simulink model "bh_4bar_model_DYN"  (R2022b)
settings: Solver=ode45  StartTime=0.0  StopTime=10  FixedStep=0.001  MaxStep=0.1  RelTol=1e-9  AbsTol=1e-9  EnableMultiTasking=on
values from neighbouring files (symbols this model uses):
  L1 = 0.4    [bh_4bar_kin_z_analysis_CLS.m]
  L2 = 1.4    [bh_4bar_kin_z_analysis_CLS.m]
  L3 = 1.2    [bh_4bar_kin_z_analysis_CLS.m]
  L4 = 1    [bh_4bar_kin_z_analysis_CLS.m]
  N = length(THE_DEG_ANG_VEC)    [bh_4bar_kin_z_analysis_CLS.m]
  X = my_stuff_T.theta_deg_vec    [bh_4bar_kin_z_analysis_CLS.m]
undefined symbols (not defined in the file or in its folder): alpha_0_rad, alpha_dot_0_rad, alpha_rad, g, H, I_G1, I_G2, I_G3, m1, m2, m3, phi_0_rad, phi_dot_0_rad, phi_rad, theta_0_rad, theta_dot_0_rad, W, Y, Z
libraries: nesl_utility x20, sm_lib x15, simulink_extras x14, bh_4bar_SL_LIB x13
(part 3 of 3)

== matlab function bh_4bar_model_DYN/Hand_model_LAG_CONSTRAINTS_invA/THE_HAND_DYN_SYS1 ==
  data: I_1 input; theta_DD output; I_2 input; I_3 input; L_1 input; L_2 input; L_3 input; alpha input; alpha_dot input; g input; m_1 input; m_2 input; m_3 input; phi input; phi_dot input; tau_1 input; theta input; theta_dot input; alpha_DD output; phi_DD output; Lambda_1 output; Lambda_2 output
function [theta_DD,alpha_DD,phi_DD,Lambda_1,Lambda_2] = THE_HAND_DYN_SYS(I_1,I_2,I_3,L_1,L_2,L_3,alpha,alpha_dot,g,m_1,m_2,m_3,phi,phi_dot,tau_1,theta,theta_dot)
%#codegen

%    This function was generated by the Symbolic Math Toolbox version 8.4.
%    11-Nov-2019 10:59:12

theta_DD = (L_2.^2.*L_3.^2.*tau_1.*4.0-L_2.^2.*L_3.^2.*tau_1.*cos(alpha.*2.0-phi.*2.0).*4.0+I_3.*L_1.^2.*L_2.^2.*theta_dot.^2.*sin(alpha.*2.0-theta.*2.0).*4.0+I_2.*L_1.^2.*L_3.^2.*theta_dot.^2.*sin(phi.*2.0-theta.*2.0).*4.0+I_3.*L_1.*L_2.^3.*alpha_dot.^2.*sin(alpha-theta).*8.0-I_2.*L_1.*L_3.^3.*phi_dot.^2.*sin(phi-theta).*8.0+L_1.^2.*L_2.^2.*L_3.^2.*m_2.*theta_dot.^2.*sin(alpha.*2.0-theta.*2.0).*2.0+L_1.^2.*L_2.^2.*L_3.^2.*m_3.*theta_dot.^2.*sin(alpha.*2.0-theta.*2.0)-L_1.^2.*L_2.^2.*L_3.^2.*m_2.*theta_dot.^2.*sin(phi.*2.0-theta.*2.0)-I_2.*L_1.*L_2.*L_3.^2.*alpha_dot.^2.*sin(alpha-phi.*2.0+theta).*4.0+L_1.*L_2.^2.*L_3.^2.*g.*m_2.*cos(alpha.*2.0-theta)+L_1.*L_2.^2.*L_3.^2.*g.*m_3.*cos(alpha.*2.0-theta)+I_3.*L_1.*L_2.^2.*L_3.*phi_dot.^2.*sin(alpha.*-2.0+phi+theta).*4.0+L_1.*L_2.^3.*L_3.^2.*alpha_dot.^2.*m_2.*sin(alpha-theta).*3.0+L_1.*L_2.^3.*L_3.^2.*alpha_dot.^2.*m_3.*sin(alpha-theta).*2.0-L_1.*L_2.^2.*L_3.^2.*g.*m_2.*cos(phi.*2.0-theta)-L_1.*L_2.^2.*L_3.^2.*g.*m_3.*cos(phi.*2.0-theta)-L_1.*L_2.^2.*L_3.^3.*m_3.*phi_dot.^2.*sin(phi-theta)+L_1.*L_2.^2.*L_3.^2.*g.*m_1.*cos(alpha.*-2.0+phi.*2.0+theta)+L_1.*L_2.^2.*L_3.^2.*g.*m_1.*cos(alpha.*2.0-phi.*2.0+theta)+L_1.*L_2.^2.*L_3.^2.*g.*m_2.*cos(alpha.*-2.0+phi.*2.0+theta).*2.0+L_1.*L_2.^2.*L_3.^2.*g.*m_2.*cos(alpha.*2.0-phi.*2.0+theta)+L_1.*L_2.^2.*L_3.^2.*g.*m_3.*cos(alpha.*-2.0+phi.*2.0+theta)+L_1.*L_2.^3.*L_3.^2.*alpha_dot.^2.*m_2.*sin(alpha-phi.*2.0+theta)-L_1.*L_2.^2.*L_3.^2.*g.*m_1.*cos(theta).*2.0-L_1.*L_2.^2.*L_3.^2.*g.*m_2.*cos(theta).*3.0-L_1.*L_2.^2.*L_3.^2.*g.*m_3.*cos(theta)+I_2.*L_1.*L_2.*L_3.^2.*alpha_dot.^2.*sin(alpha-theta).*4.0+L_1.*L_2.^2.*L_3.^3.*m_2.*phi_dot.^2.*sin(alpha.*-2.0+phi+theta).*2.0+L_1.*L_2.^2.*L_3.^3.*m_3.*phi_dot.^2.*sin(alpha.*-2.0+phi+theta)-I_3.*L_1.*L_2.^2.*L_3.*phi_dot.^2.*sin(phi-theta).*4.0)./(I_1.*L_2.^2.*L_3.^2.*4.0+I_2.*L_1.^2.*L_3.^2.*4.0+I_3.*L_1.^2.*L_2.^2.*4.0-I_1.*L_2.^2.*L_3.^2.*cos(alpha.*2.0-phi.*2.0).*4.0-I_3.*L_1.^2.*L_2.^2.*cos(alpha.*2.0-theta.*2.0).*4.0-I_2.*L_1.^2.*L_3.^2.*cos(phi.*2.0-theta.*2.0).*4.0+L_1.^2.*L_2.^2.*L_3.^2.*m_1+L_1.^2.*L_2.^2.*L_3.^2.*m_2.*3.0+L_1.^2.*L_2.^2.*L_3.^2.*m_3-L_1.^2.*L_2.^2.*L_3.^2.*m_1.*cos(alpha.*2.0-phi.*2.0)-L_1.^2.*L_2.^2.*L_3.^2.*m_2.*cos(alpha.*2.0-phi.*2.0).*2.0-L_1.^2.*L_2.^2.*L_3.^2.*m_2.*cos(alpha.*2.0-theta.*2.0).*2.0-L_1.^2.*L_2.^2.*L_3.^2.*m_3.*cos(alpha.*2.0-theta.*2.0)+L_1.^2.*L_2.^2.*L_3.^2.*m_2.*cos(phi.*2.0-theta.*2.0));
if nargout > 1
    alpha_DD = -(L_1.*L_2.*L_3.^2.*tau_1.*cos(alpha-theta).*4.0+I_1.*L_2.^2.*L_3.^2.*alpha_dot.^2.*sin(alpha.*2.0-phi.*2.0).*4.0+I_3.*L_1.^2.*L_2.^2.*alpha_dot.^2.*sin(alpha.*2.0-theta.*2.0).*4.0-I_1.*L_2.*L_3.^3.*phi_dot.^2.*sin(alpha-phi).*8.0+I_3.*L_1.^3.*L_2.*theta_dot.^2.*sin(alpha-theta).*8.0-L_1.*L_2.*L_3.^2.*tau_1.*cos(alpha-phi.*2.0+theta).*4.0-I_3.*L_1.^2.*L_2.*L_3.*phi_dot.^2.*sin(alpha+phi-theta.*2.0).*4.0+I_1.*L_1.*L_2.*L_3.^2.*theta_dot.^2.*sin(alpha-phi.*2.0+theta).*4.0-L_1.^2.*L_2.*L_3.^3.*m_1.*phi_dot.^2.*sin(alpha-phi).*2.0-L_1.^2.*L_2.*L_3.^3.*m_2.*phi_dot.^2.*sin(alpha-phi).*6.0-L_1.^2.*L_2.*L_3.^3.*m_3.*phi_dot.^2.*sin(alpha-phi)+L_1.^3.*L_2.*L_3.^2.*m_1.*theta_dot.^2.*sin(alpha-theta)+L_1.^3.*L_2.*L_3.^2.*m_2.*theta_dot.^2.*sin(alpha-theta).*6.0+L_1.^3.*L_2.*L_3.^2.*m_3.*theta_dot.^2.*sin(alpha-theta).*2.0-L_1.^2.*L_2.*L_3.^2.*g.*m_1.*cos(alpha)+L_1.^2.*L_2.*L_3.^2.*g.*m_3.*cos(alpha)+L_1.^2.*L_2.*L_3.^2.*g.*m_1.*cos(alpha-phi.*2.0+theta.*2.0)+L_1.^2.*L_2.*L_3.^2.*g.*m_2.*cos(alpha-phi.*2.0+theta.*2.0)-L_1.^2.*L_2.*L_3.^2.*g.*m_2.*cos(alpha+phi.*2.0-theta.*2.0)-L_1.^2.*L_2.*L_3.^2.*g.*m_3.*cos(alpha+phi.*2.0-theta.*2.0)-L_1.^2.*L_2.*L_3.^3.*m_2.*phi_dot.^2.*sin(alpha+phi-theta.*2.0).*2.0-L_1.^2.*L_2.*L_3.^3.*m_3.*phi_dot.^2.*sin(alpha+phi-theta.*2.0)+L_1.^3.*L_2.*L_3.^2.*m_1.*theta_dot.^2.*sin(alpha-phi.*2.0+theta)+L_1.^3.*L_2.*L_3.^2.*m_2.*theta_dot.^2.*sin(alpha-phi.*2.0+theta).*2.0-I_3.*L_1.^2.*L_2.*L_3.*phi_dot.^2.*sin(alpha-phi).*4.0+I_1.*L_1.*L_2.*L_3.^2.*theta_dot.^2.*sin(alpha-theta).*4.0+L_1.^2.*L_2.*L_3.^2.*g.*m_1.*cos(alpha-phi.*2.0)+L_1.^2.*L_2.*L_3.^2.*g.*m_2.*cos(alpha-phi.*2.0).*2.0+L_1.^2.*L_2.*L_3.^2.*g.*m_3.*cos(alpha-phi.*2.0)-L_1.^2.*L_2.*L_3.^2.*g.*m_1.*cos(alpha-theta.*2.0)-L_1.^2.*L_2.*L_3.^2.*g.*m_2.*cos(alpha-theta.*2.0).*2.0-L_1.^2.*L_2.*L_3.^2.*g.*m_3.*cos(alpha-theta.*2.0)+L_1.^2.*L_2.^2.*L_3.^2.*alpha_dot.^2.*m_1.*sin(alpha.*2.0-phi.*2.0)+L_1.^2.*L_2.^2.*L_3.^2.*alpha_dot.^2.*m_2.*sin(alpha.*2.0-phi.*2.0).*2.0+L_1.^2.*L_2.^2.*L_3.^2.*alpha_dot.^2.*m_2.*sin(alpha.*2.0-theta.*2.0).*2.0+L_1.^2.*L_2.^2.*L_3.^2.*alpha_dot.^2.*m_3.*sin(alpha.*2.0-theta.*2.0))./(I_1.*L_2.^2.*L_3.^2.*4.0+I_2.*L_1.^2.*L_3.^2.*4.0+I_3.*L_1.^2.*L_2.^2.*4.0-I_1.*L_2.^2.*L_3.^2.*cos(alpha.*2.0-phi.*2.0).*4.0-I_3.*L_1.^2.*L_2.^2.*cos(alpha.*2.0-theta.*2.0).*4.0-I_2.*L_1.^2.*L_3.^2.*cos(phi.*2.0-theta.*2.0).*4.0+L_1.^2.*L_2.^2.*L_3.^2.*m_1+L_1.^2.*L_2.^2.*L_3.^2.*m_2.*3.0+L_1.^2.*L_2.^2.*L_3.^2.*m_3-L_1.^2.*L_2.^2.*L_3.^2.*m_1.*cos(alpha.*2.0-phi.*2.0)-L_1.^2.*L_2.^2.*L_3.^2.*m_2.*cos(alpha.*2.0-phi.*2.0).*2.0-L_1.^2.*L_2.^2.*L_3.^2.*m_2.*cos(alpha.*2.0-theta.*2.0).*2.0-L_1.^2.*L_2.^2.*L_3.^2.*m_3.*cos(alpha.*2.0-theta.*2.0)+L_1.^2.*L_2.^2.*L_3.^2.*m_2.*cos(phi.*2.0-theta.*2.0));
end
if nargout > 2
    phi_DD = (L_1.*L_2.^2.*L_3.*tau_1.*cos(phi-theta).*4.0+I_1.*L_2.^2.*L_3.^2.*phi_dot.^2.*sin(alpha.*2.0-phi.*2.0).*4.0-I_2.*L_1.^2.*L_3.^2.*phi_dot.^2.*sin(phi.*2.0-theta.*2.0).*4.0-I_1.*L_2.^3.*L_3.*alpha_dot.^2.*sin(alpha-phi).*8.0-L_1.*L_2.^2.*L_3.*tau_1.*cos(alpha.*-2.0+phi+theta).*4.0+I_2.*L_1.^3.*L_3.*theta_dot.^2.*sin(phi-theta).*8.0+L_1.^2.*L_2.^2.*L_3.^2.*m_1.*phi_dot.^2.*sin(alpha.*2.0-phi.*2.0)+L_1.^2.*L_2.^2.*L_3.^2.*m_2.*phi_dot.^2.*sin(alpha.*2.0-phi.*2.0).*2.0+L_1.^2.*L_2.^2.*L_3.^2.*m_2.*phi_dot.^2.*sin(phi.*2.0-theta.*2.0)+I_2.*L_1.^2.*L_2.*L_3.*alpha_dot.^2.*sin(alpha+phi-theta.*2.0).*4.0+L_1.^2.*L_2.^2.*L_3.*g.*m_1.*cos(alpha.*2.0-phi)+L_1.^2.*L_2.^2.*L_3.*g.*m_2.*cos(alpha.*2.0-phi)-L_1.^2.*L_2.^3.*L_3.*alpha_dot.^2.*m_1.*sin(alpha-phi).*2.0-L_1.^2.*L_2.^3.*L_3.*alpha_dot.^2.*m_2.*sin(alpha-phi).*3.0+I_1.*L_1.*L_2.^2.*L_3.*theta_dot.^2.*sin(alpha.*-2.0+phi+theta).*4.0+L_1.^3.*L_2.^2.*L_3.*m_1.*theta_dot.^2.*sin(phi-theta)+L_1.^2.*L_2.^2.*L_3.*g.*m_1.*cos(alpha.*-2.0+phi+theta.*2.0)+L_1.^2.*L_2.^2.*L_3.*g.*m_2.*cos(alpha.*-2.0+phi+theta.*2.0).*2.0+L_1.^2.*L_2.^2.*L_3.*g.*m_2.*cos(alpha.*2.0+phi-theta.*2.0)+L_1.^2.*L_2.^2.*L_3.*g.*m_3.*cos(alpha.*-2.0+phi+theta.*2.0)+L_1.^2.*L_2.^2.*L_3.*g.*m_3.*cos(alpha.*2.0+phi-theta.*2.0)-L_1.^2.*L_2.^3.*L_3.*alpha_dot.^2.*m_2.*sin(alpha+phi-theta.*2.0)-L_1.^2.*L_2.^2.*L_3.*g.*m_1.*cos(phi)-L_1.^2.*L_2.^2.*L_3.*g.*m_2.*cos(phi).*3.0-L_1.^2.*L_2.^2.*L_3.*g.*m_3.*cos(phi).*2.0-I_2.*L_1.^2.*L_2.*L_3.*alpha_dot.^2.*sin(alpha-phi).*4.0+L_1.^3.*L_2.^2.*L_3.*m_1.*theta_dot.^2.*sin(alpha.*-2.0+phi+theta)+L_1.^3.*L_2.^2.*L_3.*m_2.*theta_dot.^2.*sin(alpha.*-2.0+phi+theta).*2.0+I_1.*L_1.*L_2.^2.*L_3.*theta_dot.^2.*sin(phi-theta).*4.0-L_1.^2.*L_2.^2.*L_3.*g.*m_1.*cos(phi-theta.*2.0)-L_1.^2.*L_2.^2.*L_3.*g.*m_2.*cos(phi-theta.*2.0))./(I_1.*L_2.^2.*L_3.^2.*4.0+I_2.*L_1.^2.*L_3.^2.*4.0+I_3.*L_1.^2.*L_2.^2.*4.0-I_1.*L_2.^2.*L_3.^2.*cos(alpha.*2.0-phi.*2.0).*4.0-I_3.*L_1.^2.*L_2.^2.*cos(alpha.*2.0-theta.*2.0).*4.0-I_2.*L_1.^2.*L_3.^2.*cos(phi.*2.0-theta.*2.0).*4.0+L_1.^2.*L_2.^2.*L_3.^2.*m_1+L_1.^2.*L_2.^2.*L_3.^2.*m_2.*3.0+L_1.^2.*L_2.^2.*L_3.^2.*m_3-L_1.^2.*L_2.^2.*L_3.^2.*m_1.*cos(alpha.*2.0-phi.*2.0)-L_1.^2.*L_2.^2.*L_3.^2.*m_2.*cos(alpha.*2.0-phi.*2.0).*2.0-L_1.^2.*L_2.^2.*L_3.^2.*m_2.*cos(alpha.*2.0-theta.*2.0).*2.0-L_1.^2.*L_2.^2.*L_3.^2.*m_3.*cos(alpha.*2.0-theta.*2.0)+L_1.^2.*L_2.^2.*L_3.^2.*m_2.*cos(phi.*2.0-theta.*2.0));
end
if nargout > 3
    Lambda_1 = (I_1.*I_3.*L_2.^3.*alpha_dot.^2.*cos(alpha).*3.2e+1-I_1.*I_2.*L_3.^3.*phi_dot.^2.*cos(phi).*3.2e+1+I_2.*I_3.*L_1.^3.*theta_dot.^2.*cos(theta).*3.2e+1-I_3.*L_1.*L_2.^2.*tau_1.*sin(alpha.*2.0-theta).*1.6e+1-I_2.*L_1.*L_3.^2.*tau_1.*sin(phi.*2.0-theta).*1.6e+1+I_2.*L_1.*L_3.^2.*tau_1.*sin(theta).*1.6e+1+I_3.*L_1.*L_2.^2.*tau_1.*sin(theta).*1.6e+1+I_3.*L_1.^2.*L_2.^2.*g.*m_1.*sin(alpha.*2.0).*4.0-I_1.*L_2.^2.*L_3.^2.*g.*m_2.*sin(alpha.*2.0).*4.0+I_3.*L_1.^2.*L_2.^2.*g.*m_2.*sin(alpha.*2.0).*4.0-I_1.*L_2.^2.*L_3.^2.*g.*m_3.*sin(alpha.*2.0).*4.0-L_1.^2.*L_2.^2.*L_3.^2.*g.*m_2.^2.*sin(phi.*2.0-theta.*2.0)-I_1.*I_3.*L_2.^2.*L_3.*phi_dot.^2.*cos(alpha.*2.0-phi).*1.6e+1-I_2.*L_1.^2.*L_3.^3.*m_1.*phi_dot.^2.*cos(phi).*8.0-I_1.*L_2.^2.*L_3.^3.*m_2.*phi_dot.^2.*cos(phi).*8.0-I_2.*L_1.^2.*L_3.^3.*m_2.*phi_dot.^2.*cos(phi).*3.2e+1-I_1.*L_2.^2.*L_3.^3.*m_3.*phi_dot.^2.*cos(phi).*4.0-I_2.*L_1.^2.*L_3.^3.*m_3.*phi_dot.^2.*cos(phi).*4.0+I_1.*I_3.*L_1.*L_2.^2.*theta_dot.^2.*cos(alpha.*2.0-theta).*1.6e+1+I_2.*L_1.^2.*L_3.^2.*g.*m_1.*sin(phi.*2.0).*4.0+I_1.*L_2.^2.*L_3.^2.*g.*m_2.*sin(phi.*2.0).*4.0+I_2.*L_1.^2.*L_3.^2.*g.*m_2.*sin(phi.*2.0).*8.0+I_1.*L_2.^2.*L_3.^2.*g.*m_3.*sin(phi.*2.0).*4.0+I_2.*L_1.^2.*L_3.^2.*g.*m_3.*sin(phi.*2.0).*4.0+I_2.*L_1.^3.*L_3.^2.*m_1.*theta_dot.^2.*cos(theta).*4.0+I_3.*L_1.^3.*L_2.^2.*m_1.*theta_dot.^2.*cos(theta).*4.0+I_2.*L_1.^3.*L_3.^2.*m_2.*theta_dot.^2.*cos(theta).*1.6e+1+I_2.*L_1.^3.*L_3.^2.*m_3.*theta_dot.^2.*cos(theta).*8.0-I_2.*L_1.^2.*L_3.^2.*g.*m_1.*sin(theta.*2.0).*4.0-I_3.*L_1.^2.*L_2.^2.*g.*m_1.*sin(theta.*2.0).*4.0-I_2.*L_1.^2.*L_3.^2.*g.*m_2.*sin(theta.*2.0).*8.0-I_3.*L_1.^2.*L_2.^2.*g.*m_2.*sin(theta.*2.0).*4.0-I_2.*L_1.^2.*L_3.^2.*g.*m_3.*sin(theta.*2.0).*4.0+I_1.*L_2.^3.*L_3.^2.*alpha_dot.^2.*m_2.*cos(alpha-phi.*2.0).*4.0+I_1.*I_2.*L_1.*L_3.^2.*theta_dot.^2.*cos(phi.*2.0-theta).*1.6e+1-I_3.*L_1.^2.*L_2.^3.*alpha_dot.^2.*m_2.*cos(alpha-theta.*2.0).*4.0-I_1.*L_2.^2.*L_3.^2.*g.*m_2.*sin(alpha.*2.0-phi.*2.0).*4.0-I_1.*L_2.^2.*L_3.^2.*g.*m_3.*sin(alpha.*2.0-phi.*2.0).*4.0+I_3.*L_1.^2.*L_2.^2.*g.*m_1.*sin(alpha.*2.0-theta.*2.0).*4.0+I_3.*L_1.^2.*L_2.^2.*g.*m_2.*sin(alpha.*2.0-theta.*2.0).*4.0-I_2.*L_1.^2.*L_3.^3.*m_3.*phi_dot.^2.*cos(phi-theta.*2.0).*4.0+I_2.*L_1.^2.*L_3.^2.*g.*m_1.*sin(phi.*2.0-theta.*2.0).*4.0+I_2.*L_1.^2.*L_3.^2.*g.*m_2.*sin(phi.*2.0-theta.*2.0).*8.0+I_2.*L_1.^2.*L_3.^2.*g.*m_3.*sin(phi.*2.0-theta.*2.0).*4.0-L_1.*L_2.^2.*L_3.^2.*m_2.*tau_1.*sin(alpha.*2.0-theta).*4.0-L_1.*L_2.^2.*L_3.^2.*m_3.*tau_1.*sin(alpha.*2.0-theta).*4.0+L_1.^3.*L_2.^2.*L_3.^2.*m_2.^2.*theta_dot.^2.*cos(alpha.*2.0-theta).*2.0-L_1.^3.*L_2.^2.*L_3.^2.*m_2.^2.*theta_dot.^2.*cos(phi.*2.0-theta).*2.0+I_1.*I_2.*L_2.*L_3.^2.*alpha_dot.^2.*cos(alpha).*1.6e+1+I_2.*I_3.*L_1.^2.*L_2.*alpha_dot.^2.*cos(alpha).*1.6e+1-I_1.*I_3.*L_2.^2.*L_3.*phi_dot.^2.*cos(phi).*1.6e+1-I_2.*I_3.*L_1.^2.*L_3.*phi_dot.^2.*cos(phi).*1.6e+1-I_1.*L_2.^2.*L_3.^3.*m_3.*phi_dot.^2.*cos(alpha.*2.0-phi).*4.0+I_1.*I_2.*L_1.*L_3.^2.*theta_dot.^2.*cos(theta).*1.6e+1+I_1.*I_3.*L_1.*L_2.^2.*theta_dot.^2.*cos(theta).*1.6e+1+I_3.*L_1.^3.*L_2.^2.*m_1.*theta_dot.^2.*cos(alpha.*2.0-theta).*4.0+I_3.*L_1.^3.*L_2.^2.*m_2.*theta_dot.^2.*cos(alpha.*2.0-theta).*8.0+I_1.*I_2.*L_2.*L_3.^2.*alpha_dot.^2.*cos(alpha-phi.*2.0).*1.6e+1+I_2.*I_3.*L_1.^2.*L_2.*alpha_dot.^2.*cos(alpha-theta.*2.0).*1.6e+1+I_2.*L_1.^3.*L_3.^2.*m_1.*theta_dot.^2.*cos(phi.*2.0-theta).*4.0+I_2.*L_1.^3.*L_3.^2.*m_2.*theta_dot.^2.*cos(phi.*2.0-theta).*1.6e+1+L_1.^2.*L_2.^3.*L_3.^2.*alpha_dot.^2.*m_2.^2.*cos(alpha)-L_1.^2.*L_2.^3.*L_3.^2.*alpha_dot.^2.*m_2.^2.*cos(alpha+phi.*2.0-theta.*2.0)+L_1.*L_2.^2.*L_3.^2.*m_2.*tau_1.*sin(alpha.*-2.0+phi.*2.0+theta).*4.0-I_2.*I_3.*L_1.^2.*L_3.*phi_dot.^2.*cos(phi-theta.*2.0).*1.6e+1+L_1.^2.*L_2.^2.*L_3.^3.*m_2.^2.*phi_dot.^2.*cos(alpha.*-2.0+phi+theta.*2.0).*2.0+L_1.^2.*L_2.^2.*L_3.^3.*m_2.^2.*phi_dot.^2.*cos(alpha.*2.0+phi-theta.*2.0).*2.0-L_1.^2.*L_2.^2.*L_3.^2.*g.*m_2.^2.*sin(alpha.*2.0)+L_1.^3.*L_2.^2.*L_3.^2.*m_2.^2.*theta_dot.^2.*cos(alpha.*-2.0+phi.*2.0+theta).*2.0+L_1.*L_2.^2.*L_3.^2.*m_3.*tau_1.*sin(theta).*4.0-L_1.^2.*L_2.^2.*L_3.^2.*g.*m_2.^2.*sin(alpha.*-2.0+phi.*2.0+theta.*2.0).*2.0-L_1.^2.*L_2.^2.*L_3.^2.*g.*m_2.^2.*sin(alpha.*2.0+phi.*2.0-theta.*2.0)-L_1.^2.*L_2.^2.*L_3.^3.*m_2.^2.*phi_dot.^2.*cos(phi).*4.0+L_1.^2.*L_2.^2.*L_3.^2.*g.*m_2.^2.*sin(phi.*2.0).*3.0-L_1.^3.*L_2.^2.*L_3.^2.*m_2.^2.*theta_dot.^2.*cos(theta).*2.0+L_1.^2.*L_2.^2.*L_3.^2.*g.*m_2.^2.*sin(theta.*2.0)+L_1.^2.*L_2.^3.*L_3.^2.*alpha_dot.^2.*m_2.^2.*cos(alpha-phi.*2.0)-L_1.^2.*L_2.^3.*L_3.^2.*alpha_dot.^2.*m_2.^2.*cos(alpha-theta.*2.0)+I_3.*L_1.^2.*L_2.^3.*alpha_dot.^2.*m_1.*cos(alpha).*8.0+I_1.*L_2.^3.*L_3.^2.*alpha_dot.^2.*m_2.*cos(alpha).*4.0+I_3.*L_1.^2.*L_2.^3.*alpha_dot.^2.*m_2.*cos(alpha).*1.2e+1+I_1.*L_2.^3.*L_3.^2.*alpha_dot.^2.*m_3.*cos(alpha).*8.0-L_1.^2.*L_2.^2.*L_3.^2.*g.*m_2.^2.*sin(alpha.*2.0-phi.*2.0)+L_1.^2.*L_2.^2.*L_3.^2.*g.*m_2.^2.*sin(alpha.*2.0-theta.*2.0)-L_1.^2.*L_2.^2.*L_3.^2.*g.*m_1.*m_3.*sin(alpha.*2.0-phi.*2.0)-L_1.^2.*L_2.^2.*L_3.^2.*g.*m_2.*m_3.*sin(alpha.*2.0-phi.*2.0).*2.0+L_1.^2.*L_2.^2.*L_3.^2.*g.*m_1.*m_2.*sin(alpha.*2.0-theta.*2.0)+L_1.^2.*L_2.^2.*L_3.^2.*g.*m_1.*m_3.*sin(alpha.*2.0-theta.*2.0)+L_1.^2.*L_2.^2.*L_3.^2.*g.*m_2.*m_3.*sin(alpha.*2.0-theta.*2.0)+L_1.^2.*L_2.^2.*L_3.^3.*m_2.*m_3.*phi_dot.^2.*cos(phi-theta.*2.0)-L_1.^2.*L_2.^2.*L_3.^2.*g.*m_2.*m_3.*sin(phi.*2.0-theta.*2.0)+I_2.*L_1.^2.*L_2.*L_3.^2.*alpha_dot.^2.*m_1.*cos(alpha).*4.0+I_2.*L_1.^2.*L_2.*L_3.^2.*alpha_dot.^2.*m_2.*cos(alpha).*1.2e+1+I_2.*L_1.^2.*L_2.*L_3.^2.*alpha_dot.^2.*m_3.*cos(alpha).*4.0+I_2.*L_1.^2.*L_2.*L_3.^2.*alpha_dot.^2.*m_2.*cos(alpha+phi.*2.0-theta.*2.0).*4.0+I_3.*L_1.^2.*L_2.^2.*L_3.*m_2.*phi_dot.^2.*cos(alpha.*-2.0+phi+theta.*2.0).*4.0+I_3.*L_1.^2.*L_2.^2.*L_3.*m_2.*phi_dot.^2.*cos(alpha.*2.0+phi-theta.*2.0).*4.0+I_1.*L_1.*L_2.^2.*L_3.^2.*m_2.*theta_dot.^2.*cos(alpha.*-2.0+phi.*2.0+theta).*4.0-I_3.*L_1.^2.*L_2.^2.*L_3.*m_1.*phi_dot.^2.*cos(phi).*4.0-I_3.*L_1.^2.*L_2.^2.*L_3.*m_2.*phi_dot.^2.*cos(phi).*1.2e+1-L_1.^2.*L_2.^2.*L_3.^3.*m_1.*m_3.*phi_dot.^2.*cos(alpha.*2.0-phi)-L_1.^2.*L_2.^2.*L_3.^3.*m_2.*m_3.*phi_dot.^2.*cos(alpha.*2.0-phi).*2.0+I_1.*L_1.*L_2.^2.*L_3.^2.*m_3.*theta_dot.^2.*cos(theta).*4.0+L_1.^3.*L_2.^2.*L_3.^2.*m_1.*m_2.*theta_dot.^2.*cos(alpha.*2.0-theta)+L_1.^3.*L_2.^2.*L_3.^2.*m_1.*m_3.*theta_dot.^2.*cos(alpha.*2.0-theta)+L_1.^3.*L_2.^2.*L_3.^2.*m_2.*m_3.*theta_dot.^2.*cos(alpha.*2.0-theta).*2.0+I_2.*L_1.^2.*L_2.*L_3.^2.*alpha_dot.^2.*m_1.*cos(alpha-phi.*2.0).*4.0+I_2.*L_1.^2.*L_2.*L_3.^2.*alpha_dot.^2.*m_2.*cos(alpha-phi.*2.0).*1.2e+1+I_2.*L_1.^2.*L_2.*L_3.^2.*alpha_dot.^2.*m_2.*cos(alpha-theta.*2.0).*4.0+I_2.*L_1.^2.*L_2.*L_3.^2.*alpha_dot.^2.*m_3.*cos(alpha-theta.*2.0).*4.0+I_3.*L_1.^2.*L_2.^2.*L_3.*m_2.*phi_dot.^2.*cos(phi-theta.*2.0).*4.0+L_1.^2.*L_2.^3.*L_3.^2.*alpha_dot.^2.*m_1.*m_2.*cos(alpha)+L_1.^2.*L_2.^3.*L_3.^2.*alpha_dot.^2.*m_1.*m_3.*cos(alpha).*2.0+L_1.^2.*L_2.^3.*L_3.^2.*alpha_dot.^2.*m_2.*m_3.*cos(alpha).*3.0+L_1.^2.*L_2.^2.*L_3.^3.*m_2.*m_3.*phi_dot.^2.*cos(alpha.*-2.0+phi+theta.*2.0)+L_1.^2.*L_2.^2.*L_3.^3.*m_2.*m_3.*phi_dot.^2.*cos(alpha.*2.0+phi-theta.*2.0)-L_1.^2.*L_2.^2.*L_3.^2.*g.*m_2.*m_3.*sin(alpha.*2.0)+L_1.^3.*L_2.^2.*L_3.^2.*m_1.*m_2.*theta_dot.^2.*cos(alpha.*-2.0+phi.*2.0+theta)-L_1.^2.*L_2.^2.*L_3.^2.*g.*m_1.*m_2.*sin(alpha.*-2.0+phi.*2.0+theta.*2.0)-L_1.^2.*L_2.^2.*L_3.^2.*g.*m_2.*m_3.*sin(alpha.*-2.0+phi.*2.0+theta.*2.0)-L_1.^2.*L_2.^2.*L_3.^2.*g.*m_2.*m_3.*sin(alpha.*2.0+phi.*2.0-theta.*2.0)-I_3.*L_1.^2.*L_2.^2.*L_3.*m_1.*phi_dot.^2.*cos(alpha.*2.0-phi).*4.0-I_3.*L_1.^2.*L_2.^2.*L_3.*m_2.*phi_dot.^2.*cos(alpha.*2.0-phi).*8.0-L_1.^2.*L_2.^2.*L_3.^3.*m_1.*m_2.*phi_dot.^2.*cos(phi).*2.0-L_1.^2.*L_2.^2.*L_3.^3.*m_1.*m_3.*phi_dot.^2.*cos(phi)-L_1.^2.*L_2.^2.*L_3.^3.*m_2.*m_3.*phi_dot.^2.*cos(phi).*3.0+I_1.*L_1.*L_2.^2.*L_3.^2.*m_2.*theta_dot.^2.*cos(alpha.*2.0-theta).*4.0+I_1.*L_1.*L_2.^2.*L_3.^2.*m_3.*theta_dot.^2.*cos(alpha.*2.0-theta).*4.0+L_1.^2.*L_2.^2.*L_3.^2.*g.*m_1.*m_2.*sin(phi.*2.0)+L_1.^2.*L_2.^2.*L_3.^2.*g.*m_1.*m_3.*sin(phi.*2.0)+L_1.^2.*L_2.^2.*L_3.^2.*g.*m_2.*m_3.*sin(phi.*2.0).*3.0+L_1.^3.*L_2.^2.*L_3.^2.*m_1.*m_3.*theta_dot.^2.*cos(theta)-L_1.^2.*L_2.^2.*L_3.^2.*g.*m_1.*m_3.*sin(theta.*2.0)+L_1.^2.*L_2.^3.*L_3.^2.*alpha_dot.^2.*m_1.*m_2.*cos(alpha-phi.*2.0)-L_1.^2.*L_2.^3.*L_3.^2.*alpha_dot.^2.*m_2.*m_3.*cos(alpha-theta.*2.0))./(I_1.*L_2.^2.*L_3.^2.*1.6e+1+I_2.*L_1.^2.*L_3.^2.*1.6e+1+I_3.*L_1.^2.*L_2.^2.*1.6e+1-I_1.*L_2.^2.*L_3.^2.*cos(alpha.*2.0-phi.*2.0).*1.6e+1-I_3.*L_1.^2.*L_2.^2.*cos(alpha.*2.0-theta.*2.0).*1.6e+1-I_2.*L_1.^2.*L_3.^2.*cos(phi.*2.0-theta.*2.0).*1.6e+1+L_1.^2.*L_2.^2.*L_3.^2.*m_1.*4.0+L_1.^2.*L_2.^2.*L_3.^2.*m_2.*1.2e+1+L_1.^2.*L_2.^2.*L_3.^2.*m_3.*4.0-L_1.^2.*L_2.^2.*L_3.^2.*m_1.*cos(alpha.*2.0-phi.*2.0).*4.0-L_1.^2.*L_2.^2.*L_3.^2.*m_2.*cos(alpha.*2.0-phi.*2.0).*8.0-L_1.^2.*L_2.^2.*L_3.^2.*m_2.*cos(alpha.*2.0-theta.*2.0).*8.0-L_1.^2.*L_2.^2.*L_3.^2.*m_3.*cos(alpha.*2.0-theta.*2.0).*4.0+L_1.^2.*L_2.^2.*L_3.^2.*m_2.*cos(phi.*2.0-theta.*2.0).*4.0);
end
if nargout > 4
    Lambda_2 = (I_1.*I_3.*L_2.^3.*alpha_dot.^2.*sin(alpha).*3.2e+1-I_1.*I_2.*L_3.^3.*phi_dot.^2.*sin(phi).*3.2e+1+I_2.*I_3.*L_1.^3.*theta_dot.^2.*sin(theta).*3.2e+1+I_3.*L_1.*L_2.^2.*tau_1.*cos(alpha.*2.0-theta).*1.6e+1+I_2.*L_1.*L_3.^2.*tau_1.*cos(phi.*2.0-theta).*1.6e+1+L_1.^2.*L_2.^2.*L_3.^2.*g.*m_2.^2.*3.0+I_2.*L_1.^2.*L_3.^2.*g.*m_1.*4.0+I_3.*L_1.^2.*L_2.^2.*g.*m_1.*4.0+I_1.*L_2.^2.*L_3.^2.*g.*m_2.*4.0+I_2.*L_1.^2.*L_3.^2.*g.*m_2.*8.0+I_3.*L_1.^2.*L_2.^2.*g.*m_2.*1.2e+1-I_1.*L_2.^2.*L_3.^2.*g.*m_3.*4.0-I_2.*L_1.^2.*L_3.^2.*g.*m_3.*4.0-I_2.*L_1.*L_3.^2.*tau_1.*cos(theta).*1.6e+1-I_3.*L_1.*L_2.^2.*tau_1.*cos(theta).*1.6e+1+I_3.*L_1.^2.*L_2.^3.*alpha_dot.^2.*m_1.*sin(alpha).*8.0+I_1.*L_2.^3.*L_3.^2.*alpha_dot.^2.*m_2.*sin(alpha).*4.0+I_3.*L_1.^2.*L_2.^3.*alpha_dot.^2.*m_2.*sin(alpha).*1.2e+1+I_1.*L_2.^3.*L_3.^2.*alpha_dot.^2.*m_3.*sin(alpha).*8.0-I_2.*L_1.^2.*L_3.^2.*g.*m_1.*cos(phi.*2.0).*4.0-I_1.*L_2.^2.*L_3.^2.*g.*m_2.*cos(phi.*2.0).*4.0-I_2.*L_1.^2.*L_3.^2.*g.*m_2.*cos(phi.*2.0).*8.0-I_1.*L_2.^2.*L_3.^2.*g.*m_3.*cos(phi.*2.0).*4.0-I_2.*L_1.^2.*L_3.^2.*g.*m_3.*cos(phi.*2.0).*4.0+I_2.*L_1.^2.*L_3.^2.*g.*m_1.*cos(theta.*2.0).*4.0+I_3.*L_1.^2.*L_2.^2.*g.*m_1.*cos(theta.*2.0).*4.0+I_2.*L_1.^2.*L_3.^2.*g.*m_2.*cos(theta.*2.0).*8.0+I_3.*L_1.^2.*L_2.^2.*g.*m_2.*cos(theta.*2.0).*4.0+I_2.*L_1.^2.*L_3.^2.*g.*m_3.*cos(theta.*2.0).*4.0-I_1.*I_3.*L_2.^2.*L_3.*phi_dot.^2.*sin(alpha.*2.0-phi).*1.6e+1-I_2.*L_1.^2.*L_3.^3.*m_1.*phi_dot.^2.*sin(phi).*8.0-I_1.*L_2.^2.*L_3.^3.*m_2.*phi_dot.^2.*sin(phi).*8.0-I_2.*L_1.^2.*L_3.^3.*m_2.*phi_dot.^2.*sin(phi).*3.2e+1-I_1.*L_2.^2.*L_3.^3.*m_3.*phi_dot.^2.*sin(phi).*4.0-I_2.*L_1.^2.*L_3.^3.*m_3.*phi_dot.^2.*sin(phi).*4.0+I_1.*I_3.*L_1.*L_2.^2.*theta_dot.^2.*sin(alpha.*2.0-theta).*1.6e+1-I_1.*L_2.^2.*L_3.^2.*g.*m_2.*cos(alpha.*2.0-phi.*2.0).*4.0+I_1.*L_2.^2.*L_3.^2.*g.*m_3.*cos(alpha.*2.0-phi.*2.0).*4.0+I_2.*L_1.^3.*L_3.^2.*m_1.*theta_dot.^2.*sin(theta).*4.0+I_3.*L_1.^3.*L_2.^2.*m_1.*theta_dot.^2.*sin(theta).*4.0+I_2.*L_1.^3.*L_3.^2.*m_2.*theta_dot.^2.*sin(theta).*1.6e+1+I_2.*L_1.^3.*L_3.^2.*m_3.*theta_dot.^2.*sin(theta).*8.0-I_3.*L_1.^2.*L_2.^2.*g.*m_1.*cos(alpha.*2.0-theta.*2.0).*4.0-I_3.*L_1.^2.*L_2.^2.*g.*m_2.*cos(alpha.*2.0-theta.*2.0).*1.2e+1-I_1.*L_2.^3.*L_3.^2.*alpha_dot.^2.*m_2.*sin(alpha-phi.*2.0).*4.0+I_1.*I_2.*L_1.*L_3.^2.*theta_dot.^2.*sin(phi.*2.0-theta).*1.6e+1+I_3.*L_1.^2.*L_2.^3.*alpha_dot.^2.*m_2.*sin(alpha-theta.*2.0).*4.0-I_2.*L_1.^2.*L_3.^2.*g.*m_1.*cos(phi.*2.0-theta.*2.0).*4.0-I_2.*L_1.^2.*L_3.^2.*g.*m_2.*cos(phi.*2.0-theta.*2.0).*8.0+I_2.*L_1.^2.*L_3.^2.*g.*m_3.*cos(phi.*2.0-theta.*2.0).*4.0+L_1.*L_2.^2.*L_3.^2.*m_2.*tau_1.*cos(alpha.*2.0-theta).*4.0+L_1.*L_2.^2.*L_3.^2.*m_3.*tau_1.*cos(alpha.*2.0-theta).*4.0+I_2.*L_1.^2.*L_3.^3.*m_3.*phi_dot.^2.*sin(phi-theta.*2.0).*4.0+L_1.^3.*L_2.^2.*L_3.^2.*m_2.^2.*theta_dot.^2.*sin(alpha.*2.0-theta).*2.0-L_1.^3.*L_2.^2.*L_3.^2.*m_2.^2.*theta_dot.^2.*sin(phi.*2.0-theta).*2.0+I_1.*I_2.*L_2.*L_3.^2.*alpha_dot.^2.*sin(alpha).*1.6e+1+I_2.*I_3.*L_1.^2.*L_2.*alpha_dot.^2.*sin(alpha).*1.6e+1-I_1.*I_3.*L_2.^2.*L_3.*phi_dot.^2.*sin(phi).*1.6e+1-I_2.*I_3.*L_1.^2.*L_3.*phi_dot.^2.*sin(phi).*1.6e+1-I_1.*L_2.^2.*L_3.^3.*m_3.*phi_dot.^2.*sin(alpha.*2.0-phi).*4.0+L_1.^2.*L_2.^2.*L_3.^2.*g.*m_1.*m_2+I_1.*I_2.*L_1.*L_3.^2.*theta_dot.^2.*sin(theta).*1.6e+1+I_1.*I_3.*L_1.*L_2.^2.*theta_dot.^2.*sin(theta).*1.6e+1+I_3.*L_1.^3.*L_2.^2.*m_1.*theta_dot.^2.*sin(alpha.*2.0-theta).*4.0+I_3.*L_1.^3.*L_2.^2.*m_2.*theta_dot.^2.*sin(alpha.*2.0-theta).*8.0-L_1.*L_2.^2.*L_3.^2.*m_2.*tau_1.*cos(alpha.*-2.0+phi.*2.0+theta).*4.0-I_1.*I_2.*L_2.*L_3.^2.*alpha_dot.^2.*sin(alpha-phi.*2.0).*1.6e+1-I_2.*I_3.*L_1.^2.*L_2.*alpha_dot.^2.*sin(alpha-theta.*2.0).*1.6e+1+I_2.*L_1.^3.*L_3.^2.*m_1.*theta_dot.^2.*sin(phi.*2.0-theta).*4.0+I_2.*L_1.^3.*L_3.^2.*m_2.*theta_dot.^2.*sin(phi.*2.0-theta).*1.6e+1+L_1.^2.*L_2.^2.*L_3.^2.*g.*m_2.^2.*cos(alpha.*2.0)-L_1.*L_2.^2.*L_3.^2.*m_3.*tau_1.*cos(theta).*4.0+L_1.^2.*L_2.^2.*L_3.^2.*g.*m_2.^2.*cos(alpha.*-2.0+phi.*2.0+theta.*2.0).*2.0+L_1.^2.*L_2.^2.*L_3.^2.*g.*m_2.^2.*cos(alpha.*2.0+phi.*2.0-theta.*2.0)+L_1.^2.*L_2.^3.*L_3.^2.*alpha_dot.^2.*m_2.^2.*sin(alpha)-L_1.^2.*L_2.^3.*L_3.^2.*alpha_dot.^2.*m_2.^2.*sin(alpha+phi.*2.0-theta.*2.0)-L_1.^2.*L_2.^2.*L_3.^2.*g.*m_2.^2.*cos(phi.*2.0).*3.0-L_1.^2.*L_2.^2.*L_3.^2.*g.*m_2.^2.*cos(theta.*2.0)+I_2.*I_3.*L_1.^2.*L_3.*phi_dot.^2.*sin(phi-theta.*2.0).*1.6e+1+L_1.^2.*L_2.^2.*L_3.^3.*m_2.^2.*phi_dot.^2.*sin(alpha.*-2.0+phi+theta.*2.0).*2.0+L_1.^2.*L_2.^2.*L_3.^3.*m_2.^2.*phi_dot.^2.*sin(alpha.*2.0+phi-theta.*2.0).*2.0+L_1.^3.*L_2.^2.*L_3.^2.*m_2.^2.*theta_dot.^2.*sin(alpha.*-2.0+phi.*2.0+theta).*2.0-L_1.^2.*L_2.^2.*L_3.^3.*m_2.^2.*phi_dot.^2.*sin(phi).*4.0-L_1.^2.*L_2.^2.*L_3.^2.*g.*m_2.^2.*cos(alpha.*2.0-phi.*2.0)-L_1.^3.*L_2.^2.*L_3.^2.*m_2.^2.*theta_dot.^2.*sin(theta).*2.0-L_1.^2.*L_2.^2.*L_3.^2.*g.*m_2.^2.*cos(alpha.*2.0-theta.*2.0).*3.0-L_1.^2.*L_2.^3.*L_3.^2.*alpha_dot.^2.*m_2.^2.*sin(alpha-phi.*2.0)+L_1.^2.*L_2.^3.*L_3.^2.*alpha_dot.^2.*m_2.^2.*sin(alpha-theta.*2.0)-I_3.*L_1.^2.*L_2.^2.*g.*m_1.*cos(alpha.*2.0).*4.0+I_1.*L_2.^2.*L_3.^2.*g.*m_2.*cos(alpha.*2.0).*4.0-I_3.*L_1.^2.*L_2.^2.*g.*m_2.*cos(alpha.*2.0).*4.0+I_1.*L_2.^2.*L_3.^2.*g.*m_3.*cos(alpha.*2.0).*4.0+L_1.^2.*L_2.^2.*L_3.^2.*g.*m_2.^2.*cos(phi.*2.0-theta.*2.0)-L_1.^2.*L_2.^3.*L_3.^2.*alpha_dot.^2.*m_1.*m_2.*sin(alpha-phi.*2.0)+L_1.^2.*L_2.^3.*L_3.^2.*alpha_dot.^2.*m_2.*m_3.*sin(alpha-theta.*2.0)-L_1.^2.*L_2.^2.*L_3.^2.*g.*m_2.*m_3.*cos(phi.*2.0-theta.*2.0)-L_1.^2.*L_2.^2.*L_3.^3.*m_2.*m_3.*phi_dot.^2.*sin(phi-theta.*2.0)+I_2.*L_1.^2.*L_2.*L_3.^2.*alpha_dot.^2.*m_1.*sin(alpha).*4.0+I_2.*L_1.^2.*L_2.*L_3.^2.*alpha_dot.^2.*m_2.*sin(alpha).*1.2e+1+I_2.*L_1.^2.*L_2.*L_3.^2.*alpha_dot.^2.*m_3.*sin(alpha).*4.0+I_2.*L_1.^2.*L_2.*L_3.^2.*alpha_dot.^2.*m_2.*sin(alpha+phi.*2.0-theta.*2.0).*4.0+I_3.*L_1.^2.*L_2.^2.*L_3.*m_2.*phi_dot.^2.*sin(alpha.*-2.0+phi+theta.*2.0).*4.0+I_3.*L_1.^2.*L_2.^2.*L_3.*m_2.*phi_dot.^2.*sin(alpha.*2.0+phi-theta.*2.0).*4.0+I_1.*L_1.*L_2.^2.*L_3.^2.*m_2.*theta_dot.^2.*sin(alpha.*-2.0+phi.*2.0+theta).*4.0-I_3.*L_1.^2.*L_2.^2.*L_3.*m_1.*phi_dot.^2.*sin(phi).*4.0-I_3.*L_1.^2.*L_2.^2.*L_3.*m_2.*phi_dot.^2.*sin(phi).*1.2e+1-L_1.^2.*L_2.^2.*L_3.^3.*m_1.*m_3.*phi_dot.^2.*sin(alpha.*2.0-phi)-L_1.^2.*L_2.^2.*L_3.^3.*m_2.*m_3.*phi_dot.^2.*sin(alpha.*2.0-phi).*2.0+I_1.*L_1.*L_2.^2.*L_3.^2.*m_3.*theta_dot.^2.*sin(theta).*4.0+L_1.^3.*L_2.^2.*L_3.^2.*m_1.*m_2.*theta_dot.^2.*sin(alpha.*2.0-theta)+L_1.^3.*L_2.^2.*L_3.^2.*m_1.*m_3.*theta_dot.^2.*sin(alpha.*2.0-theta)+L_1.^3.*L_2.^2.*L_3.^2.*m_2.*m_3.*theta_dot.^2.*sin(alpha.*2.0-theta).*2.0-I_2.*L_1.^2.*L_2.*L_3.^2.*alpha_dot.^2.*m_1.*sin(alpha-phi.*2.0).*4.0-I_2.*L_1.^2.*L_2.*L_3.^2.*alpha_dot.^2.*m_2.*sin(alpha-phi.*2.0).*1.2e+1-I_2.*L_1.^2.*L_2.*L_3.^2.*alpha_dot.^2.*m_2.*sin(alpha-theta.*2.0).*4.0-I_2.*L_1.^2.*L_2.*L_3.^2.*alpha_dot.^2.*m_3.*sin(alpha-theta.*2.0).*4.0-I_3.*L_1.^2.*L_2.^2.*L_3.*m_2.*phi_dot.^2.*sin(phi-theta.*2.0).*4.0+L_1.^2.*L_2.^2.*L_3.^2.*g.*m_2.*m_3.*cos(alpha.*2.0)+L_1.^2.*L_2.^2.*L_3.^2.*g.*m_1.*m_2.*cos(alpha.*-2.0+phi.*2.0+theta.*2.0)+L_1.^2.*L_2.^2.*L_3.^2.*g.*m_2.*m_3.*cos(alpha.*-2.0+phi.*2.0+theta.*2.0)+L_1.^2.*L_2.^2.*L_3.^2.*g.*m_2.*m_3.*cos(alpha.*2.0+phi.*2.0-theta.*2.0)+L_1.^2.*L_2.^3.*L_3.^2.*alpha_dot.^2.*m_1.*m_2.*sin(alpha)+L_1.^2.*L_2.^3.*L_3.^2.*alpha_dot.^2.*m_1.*m_3.*sin(alpha).*2.0+L_1.^2.*L_2.^3.*L_3.^2.*alpha_dot.^2.*m_2.*m_3.*sin(alpha).*3.0-L_1.^2.*L_2.^2.*L_3.^2.*g.*m_1.*m_2.*cos(phi.*2.0)-L_1.^2.*L_2.^2.*L_3.^2.*g.*m_1.*m_3.*cos(phi.*2.0)-L_1.^2.*L_2.^2.*L_3.^2.*g.*m_2.*m_3.*cos(phi.*2.0).*3.0+L_1.^2.*L_2.^2.*L_3.^2.*g.*m_1.*m_3.*cos(theta.*2.0)+L_1.^2.*L_2.^2.*L_3.^3.*m_2.*m_3.*phi_dot.^2.*sin(alpha.*-2.0+phi+theta.*2.0)+L_1.^2.*L_2.^2.*L_3.^3.*m_2.*m_3.*phi_dot.^2.*sin(alpha.*2.0+phi-theta.*2.0)+L_1.^3.*L_2.^2.*L_3.^2.*m_1.*m_2.*theta_dot.^2.*sin(alpha.*-2.0+phi.*2.0+theta)-I_3.*L_1.^2.*L_2.^2.*L_3.*m_1.*phi_dot.^2.*sin(alpha.*2.0-phi).*4.0-I_3.*L_1.^2.*L_2.^2.*L_3.*m_2.*phi_dot.^2.*sin(alpha.*2.0-phi).*8.0-L_1.^2.*L_2.^2.*L_3.^3.*m_1.*m_2.*phi_dot.^2.*sin(phi).*2.0-L_1.^2.*L_2.^2.*L_3.^3.*m_1.*m_3.*phi_dot.^2.*sin(phi)-L_1.^2.*L_2.^2.*L_3.^3.*m_2.*m_3.*phi_dot.^2.*sin(phi).*3.0+I_1.*L_1.*L_2.^2.*L_3.^2.*m_2.*theta_dot.^2.*sin(alpha.*2.0-theta).*4.0+I_1.*L_1.*L_2.^2.*L_3.^2.*m_3.*theta_dot.^2.*sin(alpha.*2.0-theta).*4.0+L_1.^2.*L_2.^2.*L_3.^2.*g.*m_1.*m_3.*cos(alpha.*2.0-phi.*2.0)+L_1.^2.*L_2.^2.*L_3.^2.*g.*m_2.*m_3.*cos(alpha.*2.0-phi.*2.0).*2.0+L_1.^3.*L_2.^2.*L_3.^2.*m_1.*m_3.*theta_dot.^2.*sin(theta)-L_1.^2.*L_2.^2.*L_3.^2.*g.*m_1.*m_2.*cos(alpha.*2.0-theta.*2.0)-L_1.^2.*L_2.^2.*L_3.^2.*g.*m_1.*m_3.*cos(alpha.*2.0-theta.*2.0)-L_1.^2.*L_2.^2.*L_3.^2.*g.*m_2.*m_3.*cos(alpha.*2.0-theta.*2.0))./(I_1.*L_2.^2.*L_3.^2.*1.6e+1+I_2.*L_1.^2.*L_3.^2.*1.6e+1+I_3.*L_1.^2.*L_2.^2.*1.6e+1-I_1.*L_2.^2.*L_3.^2.*cos(alpha.*2.0-phi.*2.0).*1.6e+1-I_3.*L_1.^2.*L_2.^2.*cos(alpha.*2.0-theta.*2.0).*1.6e+1-I_2.*L_1.^2.*L_3.^2.*cos(phi.*2.0-theta.*2.0).*1.6e+1+L_1.^2.*L_2.^2.*L_3.^2.*m_1.*4.0+L_1.^2.*L_2.^2.*L_3.^2.*m_2.*1.2e+1+L_1.^2.*L_2.^2.*L_3.^2.*m_3.*4.0-L_1.^2.*L_2.^2.*L_3.^2.*m_1.*cos(alpha.*2.0-phi.*2.0).*4.0-L_1.^2.*L_2.^2.*L_3.^2.*m_2.*cos(alpha.*2.0-phi.*2.0).*8.0-L_1.^2.*L_2.^2.*L_3.^2.*m_2.*cos(alpha.*2.0-theta.*2.0).*8.0-L_1.^2.*L_2.^2.*L_3.^2.*m_3.*cos(alpha.*2.0-theta.*2.0).*4.0+L_1.^2.*L_2.^2.*L_3.^2.*m_2.*cos(phi.*2.0-theta.*2.0).*4.0);
end

== matlab function bh_4bar_model_DYN/Hand_model_LAG_CONSTRAINTS_invA/CHECK_CONSTRAINTS/MATLAB Function ==
  data: L_1 input; EQ_X output; L_2 input; L_3 input; L_4 input; THETA input; ALPHA input; PHI input; EQ_Y output
function [EQ_X, EQ_Y] = fcn(L_1, L_2, L_3, L_4,THETA, ALPHA, PHI)

   EQ_X = L_1*cos(THETA) + L_2*cos(ALPHA) - L_3*cos(PHI) - L_4;
   EQ_Y = L_1*sin(THETA) + L_2*sin(ALPHA) - L_3*sin(PHI);
end

== matlab function bh_4bar_model_DYN/Hand_model_LAG_CONSTRAINTS_invA/CHECK_VELS_AGAINST_JACOBIANS/RATES_FROM_JACOBIANS ==
  data: theta_dot input; phi_dot output; theta input; phi input; alpha input; L1 input; L2 input; L3 input; alpha_dot output
function [phi_dot, alpha_dot] = LOC_calc_RATES_of_phi_alpha(theta_dot, theta, phi, alpha, L1, L2, L3)

    k = 1/(L3*L2*sin(phi)*cos(alpha) - L3*L2*cos(phi)*sin(alpha))

    A1 = [ -L2*cos(alpha),  -L2*sin(alpha);
           -L3*cos(phi),    -L3*sin(phi);   ];
       
    A2 = [-L1*sin(theta);
           L1*cos(theta) ];
       
   tmp_col   = k * A1 * A2 * theta_dot;
   
   phi_dot   = tmp_col(1);
   alpha_dot = tmp_col(2);
    
end

== matlab function bh_4bar_model_DYN/Simscape_model/CHECK_CONSTRAINTS/MATLAB Function ==
  data: L_1 input; EQ_X output; L_2 input; L_3 input; L_4 input; THETA input; ALPHA input; PHI input; EQ_Y output
function [EQ_X, EQ_Y] = fcn(L_1, L_2, L_3, L_4,THETA, ALPHA, PHI)

   EQ_X = L_1*cos(THETA) + L_2*cos(ALPHA) - L_3*cos(PHI) - L_4;
   EQ_Y = L_1*sin(THETA) + L_2*sin(ALPHA) - L_3*sin(PHI);
end

== matlab function bh_4bar_model_DYN/Hand_model_LAG_CONSTRAINTS_A_b/Hand_deriv_Lag/THE_A_b_HAND_DYN_SYS ==
  data: I_1 input; A output; I_2 input; I_3 input; L_1 input; L_2 input; L_3 input; alpha input; alpha_dot input; g input; m_1 input; m_2 input; m_3 input; phi input; phi_dot input; tau_1 input; theta input; theta_dot input; b output
function [A,b] = THE_A_b_HAND_DYN_SYS(I_1,I_2,I_3,L_1,L_2,L_3,alpha,alpha_dot,g,m_1,m_2,m_3,phi,phi_dot,tau_1,theta,theta_dot)
%#codegen

%    This function was generated by the Symbolic Math Toolbox version 9.2.
%    27-Oct-2022 13:46:11

A = reshape([I_1+(L_1.^2.*m_1)./4.0+L_1.^2.*m_2,(L_1.*L_2.*m_2.*cos(alpha-theta))./2.0,0.0,L_1.*sin(theta),-L_1.*cos(theta),(L_1.*L_2.*m_2.*cos(alpha-theta))./2.0,I_2+(L_2.^2.*m_2)./4.0,0.0,L_2.*sin(alpha),-L_2.*cos(alpha),0.0,0.0,I_3+(L_3.^2.*m_3)./4.0,-L_3.*sin(phi),L_3.*cos(phi),L_1.*sin(theta),L_2.*sin(alpha),-L_3.*sin(phi),0.0,0.0,-L_1.*cos(theta),-L_2.*cos(alpha),L_3.*cos(phi),0.0,0.0],[5,5]);
if nargout > 1
    b = [tau_1-g.*((L_1.*m_1.*cos(theta))./2.0+L_1.*m_2.*cos(theta))+(L_1.*L_2.*alpha_dot.*m_2.*theta_dot.*sin(alpha-theta))./2.0+(L_1.*L_2.*alpha_dot.*m_2.*sin(alpha-theta).*(alpha_dot-theta_dot))./2.0;L_2.*g.*m_2.*cos(alpha).*(-1.0./2.0)-(L_1.*L_2.*alpha_dot.*m_2.*theta_dot.*sin(alpha-theta))./2.0+(L_1.*L_2.*m_2.*theta_dot.*sin(alpha-theta).*(alpha_dot-theta_dot))./2.0;L_3.*g.*m_3.*cos(phi).*(-1.0./2.0);-L_2.*alpha_dot.^2.*cos(alpha)+L_3.*phi_dot.^2.*cos(phi)-L_1.*theta_dot.^2.*cos(theta);-L_2.*alpha_dot.^2.*sin(alpha)+L_3.*phi_dot.^2.*sin(phi)-L_1.*theta_dot.^2.*sin(theta)];
end
